simulink model "simulink_model_discrete"  (R2024a)
settings: Solver=VariableStepAuto  StartTime=0.0  StopTime=30  RelTol=1e-3
libraries: simulink x1
settings Model: Creator=hp  LastModifiedBy=hp

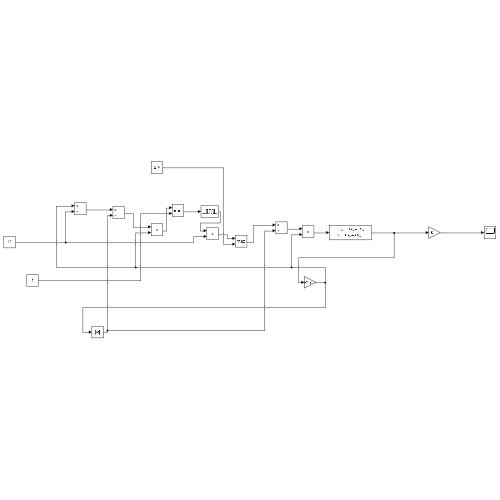
[thumbnail: Simulink's stored preview of the top-level diagram]
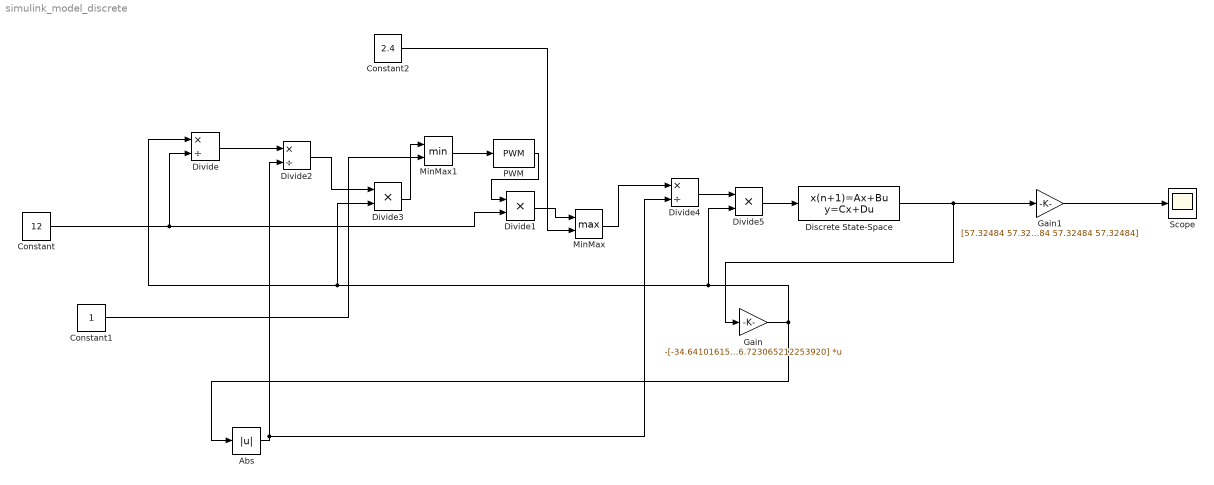
== system simulink_model_discrete ==
  Abs : Abs  SaturateOnIntegerOverflow=off
  Constant : Constant  Value=12
  Constant1 : Constant
  Constant2 : Constant  Value=2.4
  Discrete State-Space : DiscreteStateSpace  A=|  B=|  C=eye(4)  D=[0;0;0;0]  InitialCondition=[0.25; 0.035; 0; 0]  SampleTime=0.001
      A=|
      | [[1	6.19575828137124e-05	0.000999211806026587	2.06551649026597e-08];
      | [0	1.00005579723417	-3.62444285281233e-07	0.00100001860025693];
      | [0	0.123883753565288	0.998424018838491	6.19575828137124e-05];
      | [0	0.111580531720207	-0.000724704813839022	1.00005579723417]]
      B=|
      | [2.81799775979057e-05;
      | 1.29583226771982e-05;
      | 0.0563454115662880;
      | 0.0259100755752243]
  Divide : Product  Inputs=*/
  Divide1 : Product  Inputs=**
  Divide2 : Product  Inputs=*/
  Divide3 : Product  Inputs=**
  Divide4 : Product  Inputs=*/
  Divide5 : Product  Inputs=**
  Gain : Gain  Gain=-[-34.641016151376206,3.424425469457670e+02,-14.767527570011810,46.723065212253920]  Multiplication=Matrix(K*u)
  Gain1 : Gain  Gain=[57.32484 57.32484 57.32484 57.32484]
  MinMax : MinMax  Function=max  Inputs=2  OutMin=2.4  OutMax=12
  MinMax1 : MinMax  Inputs=2  OutMin=0  OutMax=1
  PWM : simulink/Discontinuities/PWM  DisableCoverage=on  Period=0.001  InitialDelay=0  DisallowZeroDutyCycle=off  RunAtFixedTimeIntervals=off  SampleTime=0.1
  Scope : Scope
  wires:
  Discrete State-Space/1 -> Gain1/1, Gain/1
  Gain/1 -> Abs/1, Divide5/2, Divide3/2, Divide/1
  Divide4/1 -> Divide5/1
  MinMax/1 -> Divide4/1
  Divide2/1 -> Divide3/1
  Divide/1 -> Divide2/1
  Constant/1 -> Divide1/2, Divide/2
  Divide1/1 -> MinMax/1
  PWM/1 -> Divide1/1
  Divide5/1 -> Discrete State-Space/1
  Abs/1 -> Divide4/2, Divide2/2
  Gain1/1 -> Scope/1
  Divide3/1 -> MinMax1/1
  MinMax1/1 -> PWM/1
  Constant1/1 -> MinMax1/2
  Constant2/1 -> MinMax/2
